simulink model "optimpid_model"  (Simulink 10.1)
settings: Solver=ode4  StartTime=0.0  StopTime=stop_time  FixedStep=step_time  RelTol=1e-3
InitFcn:
  | m = 1   ; % ball weight (kg)
  | d = 0.05; % gear rediuce (m)
  | a = 0.02; % ball rediuce (m)
  | L = 1   ; % bar length (m)
  | g = 9.8 ; % m/s^2
undefined symbols (not defined in the file or in its folder): den_G_R_V, den_st, num_G_R_V, num_st
settings Model: Creator=Ali  LastModifiedBy=msi
settings DataIOCC: SaveFormat=Dataset  ReturnWorkspaceOutputs=on
settings OptimizationCC: LifeSpan=auto
settings DebuggingCC: UnderspecifiedInitializationDetection=Simplified  MergeDetectMultiDrivingBlocksExec=error  SFUnexpectedBacktrackingDiag=error  SFNoUnconditionalDefaultTransitionDiag=error  SFExecutionAtInitializationDiag=warning  ArithmeticOperatorsInVariantConditions=error
settings HardwareCC: ProdBitPerPointer=64  ProdBitPerSizeT=64  ProdBitPerPtrDiffT=64  ProdLargestAtomicFloat=Float  ProdIntDivRoundTo=Zero  ProdEndianess=LittleEndian  ProdWordSize=64  ProdHWDeviceType=Intel->x86-64 (Windows64)
settings ModelReferenceCC: PropagateSignalLabelsOutOfModel=on
settings SFSimCC: SimUseLocalCustomCode=on  CustomCodeUndefinedFunction=FilterOut
settings RTWCC: RTWUseLocalCustomCode=on
settings CodeAppCC: StateflowObjectComments=off
settings GRTTargetCC: TargetLangStandard=C99 (ISO)  CombineOutputUpdateFcns=on  GRTInterface=off
settings ConfigComp: CovMetricSettings=dwe  CovHtmlReporting=off  CovSaveCumulativeToWorkspaceVar=off  CovSaveSingleToWorkspaceVar=off  CovExternalEMLEnable=on

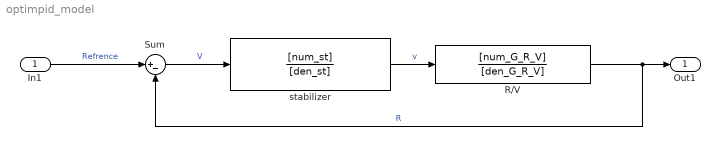
== system optimpid_model ==
  In1 : Inport
  R/V : TransferFcn  Numerator=[num_G_R_V]  Denominator=[den_G_R_V]
  Sum : Sum  Inputs=|+-
  stabilizer : TransferFcn  Numerator=[num_st]  Denominator=[den_st]
  Out1 : Outport
  wires:
  In1/1 -> Sum/1  "Refrence"
  stabilizer/1 -> R/V/1  "v"
  R/V/1 -> Sum/2, Out1/1  "R"
  Sum/1 -> stabilizer/1  "V"
